simulink model "Autopilot_q_full_5may_new"  (R2020a)
settings: Solver=ode4  StartTime=0.0  StopTime=300  FixedStep=0.01  RelTol=1e-3
undefined symbols (not defined in the file or in its folder): Aero_cofficients, Atmosphere_pert, Atmospheric_model, Counter_sensor_model, Earth, error_global, flags_global, Guidance_Flags_global, INT_global, param_guidance, Payload_data, Plane_state_mode_finish_catcher_ftr_mode, Plane_state_mode_finish_catcher_fw_mode, Plane_state_mode_finish_catcher_q_mode, Plane_state_mode_finish_catcher_rtr_mode, Plane_state_store, propulsion_model, propulsion_model_int, Structural_data, Thrust_data_store, time_global, WGS84, Wind_data, Wind_model_int, Wind_pert_factor
libraries: simulink x33, aerolibactuator x15, cstblocks x3, aerolibatmos2 x2, aerolibfltsims x1, aerolibtransform2 x1, shared6dof x1
(part 7 of 10)

== matlab function Autopilot_q_full_5may_new/GUIDANCE/    MODE SWITCHER   &   PATH PLANNER   ==
  data: Time_global input; flags_global input; u_dot_d output; v_dot_d output; t input; Plane_state input; w_dot_d output; flags_global output; param_guidance output; param_guidance input; guidance_global input; INT_global input; error_global input; guidance_global output; INT_global output; error_global output; Wind_ned input; propulsion_data input; atmos_data input; wind_pert_factor input; propulsion_pert_factor input; structure_pert_factor input; atmos_pert_factor input; aero_coff_pert_factor input; data7 input; data8 input; data9 input; data10 input; data11 input; data12 input
function [u_dot_d,v_dot_d,w_dot_d,flags_global, param_guidance,guidance_global,INT_global,error_global] = fcn(Time_global, flags_global, t, Plane_state,param_guidance,guidance_global,INT_global,error_global, Wind_ned, propulsion_data, atmos_data, wind_pert_factor, propulsion_pert_factor, structure_pert_factor, atmos_pert_factor, aero_coff_pert_factor, data7, data8, data9, data10, data11, data12)

u_dot_d=0.0;
v_dot_d=0.0;
w_dot_d=0.0;

X_i_takeoff=guidance_global(1);  Y_i_takeoff=guidance_global(2);  Z_i_takeoff=guidance_global(3); X_f_takeoff=guidance_global(4); Y_f_takeoff=guidance_global(5); Z_f_takeoff=guidance_global(6);

X_i_hover=guidance_global(7); Y_i_hover=guidance_global(8); Z_i_hover=guidance_global(9); X_f_hover=guidance_global(10); Y_f_hover=guidance_global(11); Z_f_hover=guidance_global(12);

X_i_cruise=guidance_global(13); Y_i_cruise=guidance_global(14); Z_i_cruise=guidance_global(15); X_f_cruise=guidance_global(16); Y_f_cruise=guidance_global(17); Z_f_cruise=guidance_global(18);

X_i_circle=guidance_global(19); Y_i_circle=guidance_global(20); Z_i_circle=guidance_global(21); X_f_circle=guidance_global(22); Y_f_circle=guidance_global(23); Z_f_circle=guidance_global(24);

X_i_landing=guidance_global(25); Y_i_landing=guidance_global(26); Z_i_landing=guidance_global(27); X_f_landing=guidance_global(28); Y_f_landing=guidance_global(29); Z_f_landing=guidance_global(30);

X_f_forward_transition=guidance_global(31); Y_f_forward_transition=guidance_global(32); Z_f_forward_transition=guidance_global(33);

X_i_forward_transition=guidance_global(37); Y_i_forward_transition=guidance_global(38); Z_i_forward_transition=guidance_global(39);

X_f_reverse_transition=guidance_global(43); Y_f_reverse_transition=guidance_global(44); Z_f_reverse_transition=guidance_global(45);

X_i_reverse_transition=guidance_global(49); Y_i_reverse_transition=guidance_global(50); Z_i_reverse_transition=guidance_global(51);

INT_X=INT_global(1); INT_Y=INT_global(2); INT_Z=INT_global(3);

INT_vx=INT_global(4); INT_vy=INT_global(5); INT_vz=INT_global(6);

INT_phi=INT_global(7); INT_theta=INT_global(8); INT_psi=INT_global(9);

INT_p=INT_global(10); INT_q=INT_global(11); INT_r=INT_global(12);

INT_alpha=INT_global(13); INT_beta=INT_global(14);

R_circ=param_guidance(1);
cruise_speed=param_guidance(2);

lmt_pos=param_guidance(3); lmt_vel=param_guidance(4);


error_X_old=error_global(1); error_Y_old=error_global(2); error_Z_old=error_global(3);

error_vx_old=error_global(4); error_vy_old=error_global(5); error_vz_old=error_global(6);





limit_position_X=0.001;
limit_position_Y=0.001;
limit_position_Z=0.001;
limit_velocity_vx=0.001;
limit_velocity_vy=0.001;
limit_velocity_vz=0.001;

tf0=Time_global(1);
%% Initial lift off hover
tf1=Time_global(2);
%% Vertical Takeoff
tf2=Time_global(3);
%% Hover
tf3=Time_global(4);
%% Transition Forward
tf4=Time_global(5);
%% Cruise/circle or Fixed wing mode
tf5=Time_global(6);
%% Reverse Transition
tf6=Time_global(7);
%% Hover
tf7=Time_global(8);
%% Vertical Land
tf8 = Time_global(9);
%%

all_initial_check_ok=flags_global(1);
default_mode=flags_global(2);
quad_mode=flags_global(3);
Transition_mode=flags_global(4);
Fixed_wing_mode=flags_global(5);
fail_safe_mode=flags_global(6);
fail_safe_mode_hover=flags_global(7);
fail_safe_mode_land=flags_global(8);
fail_safe_mode_2=flags_global(9);
flag_initial_lift_off_hover = flags_global(10);
flag_vertical_takeoff = flags_global(11);
flag_hover_mode = flags_global(12);
flag_circle_mode =  flags_global(13);
flag_cruise_mode = flags_global(14);
flag_vertical_landing = flags_global(15);

one_time_initial_lift_off_hover = flags_global(16);
one_time_initial_vertical_takeoff = flags_global(17);
one_time_initial_hover_mode = flags_global(18);
one_time_initial_cruise_mode = flags_global(19);
one_time_initial_circle_mode = flags_global(20);
one_time_initial_vertical_landing = flags_global(21);

flag_brake_mode=flags_global(22);

flag_forward_transition=flags_global(23);
flag_reverse_transition=flags_global(24);

one_time_initial_flag_forward_transition = flags_global(25);
one_time_initial_flag_reverse_transition = flags_global(26);


if ((t>=tf0)&&(t<tf1))
    quad_mode=1;
    Transition_mode=0;
    Fixed_wing_mode=0;
    flag_initial_lift_off_hover=1;
    flag_vertical_takeoff=0;
    flag_hover_mode=0;
    flag_cruise_mode=0;
    flag_circle_mode=0;
    flag_vertical_landing=0;
    flag_forward_transition=0;
    flag_reverse_transition=0;
    flag_brake_mode=0;
   % one_time_initial_lift_off_hover = 1;
    one_time_initial_vertical_takeoff =1;
    one_time_initial_hover_mode = 1;
    one_time_initial_cruise_mode = 1;
    one_time_initial_circle_mode = 1;
    one_time_initial_vertical_landing =1;
    one_time_initial_flag_forward_transition = 1;
    one_time_initial_flag_reverse_transition =1 ;

    
end

if ((t>=tf1)&&(t<tf2))
    quad_mode=1;
    Transition_mode=0;
    Fixed_wing_mode=0;
    flag_initial_lift_off_hover=0;
    flag_vertical_takeoff=1;
    flag_hover_mode=0;
    flag_cruise_mode=0;
    flag_circle_mode=0;
    flag_vertical_landing=0;
    flag_forward_transition=0;
    flag_reverse_transition=0;
    flag_brake_mode=0;
    one_time_initial_lift_off_hover = 1;
    %one_time_initial_vertical_takeoff =1;
    one_time_initial_hover_mode = 1;
    one_time_initial_cruise_mode = 1;
    one_time_initial_circle_mode = 1;
    one_time_initial_vertical_landing =1;
    one_time_initial_flag_forward_transition = 1;
    one_time_initial_flag_reverse_transition =1 ;
end

if ((t>=tf2)&&(t<tf3))
    quad_mode=1;
    Transition_mode=0;
    Fixed_wing_mode=0;
    flag_initial_lift_off_hover=0;
    flag_vertical_takeoff=0;
    flag_hover_mode=1;
    flag_cruise_mode=0;
    flag_circle_mode=0;
    flag_vertical_landing=0;
    flag_forward_transition=0;
    flag_reverse_transition=0;
    flag_brake_mode=0;
    one_time_initial_lift_off_hover = 1;
    one_time_initial_vertical_takeoff =1;
    %one_time_initial_hover_mode = 1;
    one_time_initial_cruise_mode = 1;
    one_time_initial_circle_mode = 1;
    one_time_initial_vertical_landing =1;
    one_time_initial_flag_forward_transition = 1;
    one_time_initial_flag_reverse_transition =1 ;
end

if ((t>=tf3)&&(t<tf4))
    quad_mode=0;
    Transition_mode=1;
    Fixed_wing_mode=0;
    flag_forward_transition=1;
    flag_reverse_transition=0;
    flag_initial_lift_off_hover=0;
    flag_vertical_takeoff=0;
    flag_hover_mode=0;
    flag_cruise_mode=0;
    flag_circle_mode=0;
    flag_vertical_landing=0;
    flag_brake_mode=0;
    one_time_initial_lift_off_hover = 1;
    one_time_initial_vertical_takeoff =1;
    one_time_initial_hover_mode = 1;
    one_time_initial_cruise_mode = 1;
    one_time_initial_circle_mode = 1;
    one_time_initial_vertical_landing =1;
    %one_time_initial_flag_forward_transition = 1;
    one_time_initial_flag_reverse_transition =1 ;
end

if ((t>=tf4)&&(t<tf5))
    quad_mode=0;
    Transition_mode=0;
    Fixed_wing_mode=1;
    flag_cruise_mode=1;
    flag_circle_mode=0;
    flag_initial_lift_off_hover=0;
    flag_vertical_takeoff=0;
    flag_hover_mode=0;
    flag_vertical_landing=0;
    flag_forward_transition=0;
    flag_reverse_transition=0;
    flag_brake_mode=0;
    one_time_initial_lift_off_hover = 1;
    one_time_initial_vertical_takeoff =1;
    one_time_initial_hover_mode = 1;
    %one_time_initial_cruise_mode = 1;
    one_time_initial_circle_mode = 1;
    one_time_initial_vertical_landing =1;
    one_time_initial_flag_forward_transition = 1;
    one_time_initial_flag_reverse_transition =1 ;
end

if ((t>=tf5)&&(t<tf6))
    quad_mode=0;
    Transition_mode=1;
    Fixed_wing_mode=0;
    flag_forward_transition=0;
    flag_reverse_transition=1;
    flag_initial_lift_off_hover=0;
    flag_vertical_takeoff=0;
    flag_hover_mode=0;
    flag_cruise_mode=0;
    flag_circle_mode=0;
    flag_vertical_landing=0;
    flag_brake_mode=0;
    one_time_initial_lift_off_hover = 1;
    one_time_initial_vertical_takeoff =1;
    one_time_initial_hover_mode = 1;
    one_time_initial_cruise_mode = 1;
    one_time_initial_circle_mode = 1;
    one_time_initial_vertical_landing =1;
    one_time_initial_flag_forward_transition = 1;
   % one_time_initial_flag_reverse_transition =1 ;

end

if ((t>=tf6)&&(t<tf7))
    quad_mode=1;
    Transition_mode=0;
    Fixed_wing_mode=0;
    flag_initial_lift_off_hover=0;
    flag_vertical_takeoff=0;
    flag_hover_mode=1;
    flag_cruise_mode=0;
    flag_circle_mode=0;
    flag_vertical_landing=0;
    flag_forward_transition=0;
    flag_reverse_transition=0;
    flag_brake_mode=0;
    %one_time_initial_lift_off_hover = 1;
    one_time_initial_vertical_takeoff =1;
    one_time_initial_hover_mode = 1;
    one_time_initial_cruise_mode = 1;
    one_time_initial_circle_mode = 1;
    one_time_initial_vertical_landing =1;
    one_time_initial_flag_forward_transition = 1;
    one_time_initial_flag_reverse_transition =1 ;
end

if ((t>=tf7)&&(t<tf8))
    quad_mode=1;
    Transition_mode=0;
    Fixed_wing_mode=0;
    flag_initial_lift_off_hover=0;
    flag_vertical_takeoff=0;
    flag_hover_mode=0;
    flag_cruise_mode=0;
    flag_circle_mode=0;
    flag_vertical_landing=1;
    flag_forward_transition=0;
    flag_reverse_transition=0;
    flag_brake_mode=0;
    one_time_initial_lift_off_hover = 1;
    one_time_initial_vertical_takeoff =1;
    one_time_initial_hover_mode = 1;
    one_time_initial_cruise_mode = 1;
    one_time_initial_circle_mode = 1;
    %one_time_initial_vertical_landing =1;
    one_time_initial_flag_forward_transition = 1;
    one_time_initial_flag_reverse_transition =1 ;
end

u=Plane_state(1);
v=Plane_state(2);
w=Plane_state(3);
p=Plane_state(4);
q=Plane_state(5);
r=Plane_state(6);
phi=Plane_state(7);
theta=Plane_state(8);
psi=Plane_state(9);
X=Plane_state(10);
Y=Plane_state(11);
Z=Plane_state(12);

R_v_v1=[cos(psi) sin(psi) 0; -sin(psi) cos(psi) 0; 0 0 1];
R_v1_v2=[cos(theta) 0 -sin(theta) ;0 1 0; sin(theta) 0 cos(theta)];
R_v2_b=[1 0 0;0 cos(phi) sin(phi) ;0 -sin(phi) cos(phi)];
R_v_b=R_v2_b*R_v1_v2*R_v_v1;



V_wind_bd=R_v_b*[Wind_ned(1);Wind_ned(2);Wind_ned(3)];

ppp = [u-V_wind_bd(1); v; w];
u_r=ppp(1);
v_r=ppp(2);
w_r=ppp(3);

V=sqrt(u_r^2+v_r^2+w_r^2);


%%
%%%%%%%%%%%%%%%%%%%%%%%%%%%%%%%%%%%%%%%%%%%%%%%%%%%%%%%%%%%%%%%%%%%%%%%%%%%%%%%%%%%%%%%%%%%%%%%%%%%%%%%%%%%%%%%%%%%%%%%%%%%%
%%%%%%%%%%%%%%%%%%%%%%%%%%%%%%%%%%%%%%%%%%%%%%%%%%%%%%%%%%%%%%%%%%%%%%%%%%%%%%%%%%%%%%%%%%%%%%%%%%%%%%%%%%%%%%%%%%%%%%%%%%%%
%%%%%%%%%%%%%%%%%%%%%%%%%%%%%%%%%%%%%%%%%%%%%%%%%%%%%%%%%%%%%%%%%%%%%%%%%%%%%%%%%%%%%%%%%%%%%%%%%%%%%%%%%%%%%%%%%%%%%%%%%%%%
if (default_mode==1)
    X_d=X;
    Y_d=Y;
    Z_d=Z;
    u_d=0.0;
    v_d=0.0;
    w_d=0.0;
    
    
    Kp_vx= 0.1*4.0*3.0;  
    Kp_vy= 0.1*4.0*3.0;    
    Kp_vz= 6.0;            
    
    error_vx = (u_d-u);
    error_vy = (v_d-v);
    error_vz = (w_d-w);
    
    u_dot_d = Kp_vx*(error_vx) ;  
    v_dot_d = Kp_vy*(error_vy) ;
    w_dot_d = Kp_vz*(error_vz) ;
end
%%
if (fail_safe_mode==0)
    
if (flag_initial_lift_off_hover==1)
    if (one_time_initial_hover_mode==1)
        X_i_hover=X;
        Y_i_hover=Y;
        Z_i_hover=Z;
        
        X_f_hover=X_i_hover;
        Y_f_hover=Y_i_hover;
        Z_f_hover=Z_i_hover;
        
        INT_X=0;INT_Y=0;INT_Z=0;
        INT_vx=0;INT_vy=0;INT_vz=0;
        INT_alpha=0;INT_beta=0;
        
        INT_phi=0;INT_theta=0;INT_psi=0;
        INT_p=0;INT_q=0;INT_r=0;
        
        one_time_initial_hover_mode=0;
    end
    
    X_d=X_f_hover;
    Y_d=Y_f_hover;
    Z_d=Z_f_hover;
    
    Kp_X=0.1*2.0;           Ki_X= 0.0;                Kd_X=0.0;
    Kp_Y=0.1*2.0;           Ki_Y= 0.0;                Kd_Y=0.0;
    Kp_Z=0.1;               Ki_Z=Kp_Z/10.0;           Kd_Z=0.0;
    
    Kp_vx= 0.1*2.0*3.0;     Ki_vx=0.0;                Kd_vx=0.0;
    Kp_vy= 0.1*2.0*3.0;     Ki_vy=0.0;                Kd_vy=0.0;
    Kp_vz= 0.3;             Ki_vz=0.01;               Kd_vz=0.0;
    
    
    error_X = (X_d-X);
    error_Y = (Y_d-Y);
    error_Z = (Z_d-Z);
    
    if(lmt_pos==1)
        
        if(abs(error_X)<limit_position_X)
            
            error_X=0.0;
        end
        if(abs(error_Y)<limit_position_Y)
            
            error_Y=0.0;
        end
        if(abs(error_Z)<limit_position_Z)
            
            error_Z=0.0;
        end
    end
    
    INT_X = INT_X + 0.01*(error_X);
    INT_Y = INT_Y + 0.01*(error_Y);
    INT_Z = INT_Z + 0.01*(error_Z);
    
    U_d = Kp_X*(error_X) +  Ki_X*(INT_X) + Kd_X*(error_X-error_X_old);
    V_d = Kp_Y*(error_Y) +  Ki_Y*(INT_Y) + Kd_Y*(error_Y-error_Y_old);
    W_d = Kp_Z*(error_Z) +  Ki_Z*(INT_Z) + Kd_Z*(error_Z-error_Z_old);
    
    temp_3X1=R_v_b*[U_d;V_d;W_d];
    
    u_d=temp_3X1(1);
    v_d=temp_3X1(2);
    w_d=temp_3X1(3);
    
    error_X_old=error_X;
    error_Y_old=error_Y;
    error_Z_old=error_Z;
    
    error_vx = (u_d-u);
    error_vy = (v_d-v);
    error_vz = (w_d-w);
    
    if(lmt_vel==1)
        if(abs(error_vx)<limit_velocity_vx)
            error_vx=0.0;
        end
        if(abs(error_vy)<limit_velocity_vy)
            error_vy=0.0;
        end
        if(abs(error_vz)<limit_velocity_vz)
            error_vz=0.0;
        end
    end
    
    INT_vx= INT_vx + 0.01*(error_vx);
    INT_vy= INT_vy + 0.01*(error_vy);
    INT_vz= INT_vz + 0.01*(error_vz);
    
    u_dot_d = Kp_vx*(error_vx)   +    Ki_vx*(INT_vx)  +   Kd_vx*(error_vx-error_vx_old);
    v_dot_d = Kp_vy*(error_vy)   +    Ki_vy*(INT_vy)  +   Kd_vy*(error_vy-error_vy_old);
    w_dot_d = Kp_vz*(error_vz)   +    Ki_vz*(INT_vz)  +   Kd_vz*(error_vz-error_vz_old);
    
    error_vx_old=error_vx;
    error_vy_old=error_vy;
    error_vz_old=error_vz;
    
end

if (flag_vertical_takeoff==1)
    if (one_time_initial_vertical_takeoff==1)
        
        X_i_takeoff = X;
        Y_i_takeoff = Y;
        Z_i_takeoff = Z;
        
        X_f_takeoff = X_i_takeoff;
        Y_f_takeoff = Y_i_takeoff;
        Z_f_takeoff = Z_i_takeoff-50.0;
        
        INT_X=0;INT_Y=0;INT_Z=0;
        INT_vx=0;INT_vy=0;INT_vz=0;
        
        INT_alpha=0;INT_beta=0;
        
        INT_phi=0;INT_theta=0;INT_psi=0;
        INT_p=0;INT_q=0;INT_r=0;
        
        one_time_initial_vertical_takeoff=0;
        one_time_initial_hover_mode=1;
    end
    
    X_d=X_f_takeoff;
    Y_d=Y_f_takeoff;
    Z_d=Z_i_takeoff + 2*(Z_f_takeoff-Z_i_takeoff)*(t-tf1)/(tf2-tf1) +(Z_i_takeoff-Z_f_takeoff)*((t-tf1)^2)/((tf2-tf1)^2) ;
   if t>tf2
       Z_d = Z_f_takeoff;
    end
    Kp_X=0.1*4.0;           Ki_X= 0.0;                Kd_X=0.0;
    Kp_Y=0.1*4.0;           Ki_Y= 0.0;                Kd_Y=0.0;
    Kp_Z=2.0;              Ki_Z=0.1;           Kd_Z=0.0;
    
    Kp_vx= 0.1*4.0*3.0;     Ki_vx=0.0;                Kd_vx=0.0;
    Kp_vy= 0.1*4.0*3.0;     Ki_vy=0.0;                Kd_vy=0.0;
    Kp_vz= 6.0;             Ki_vz=0.0*0.001;               Kd_vz=0.0;
    
    
    error_X = (X_d-X);
    error_Y = (Y_d-Y);
    error_Z = (Z_d-Z);
    
    if(lmt_pos==1)
        
        if(abs(error_X)<limit_position_X)
            
            error_X=0.0;
        end
        if(abs(error_Y)<limit_position_Y)
            
            error_Y=0.0;
        end
        if(abs(error_Z)<limit_position_Z)
            
            error_Z=0.0;
        end
    end
    
    INT_X = INT_X + 0.01*(error_X);
    INT_Y = INT_Y + 0.01*(error_Y);
    INT_Z = INT_Z + 0.01*(error_Z);
    
    U_d = Kp_X*(error_X) +  Ki_X*(INT_X) + Kd_X*(error_X-error_X_old);
    V_d = Kp_Y*(error_Y) +  Ki_Y*(INT_Y) + Kd_Y*(error_Y-error_Y_old);
    W_d = Kp_Z*(error_Z) +  Ki_Z*(INT_Z) + Kd_Z*(error_Z-error_Z_old);
    
    temp_3X1=R_v_b*[U_d;V_d;W_d];
    
    u_d=temp_3X1(1);
    v_d=temp_3X1(2);
    w_d=temp_3X1(3);
    error_X_old=error_X;
    error_Y_old=error_Y;
    error_Z_old=error_Z;
    
    error_vx = (u_d-u);
    error_vy = (v_d-v);
    error_vz = (w_d-w);
    
    if(lmt_vel==1)
        if(abs(error_vx)<limit_velocity_vx)
            error_vx=0.0;
        end
        if(abs(error_vy)<limit_velocity_vy)
            error_vy=0.0;
        end
        if(abs(error_vz)<limit_velocity_vz)
            error_vz=0.0;
        end
    end
    
    INT_vx= INT_vx + 0.01*(error_vx);
    INT_vy= INT_vy + 0.01*(error_vy);
    INT_vz= INT_vz + 0.01*(error_vz);
    
    u_dot_d = Kp_vx*(error_vx)   +    Ki_vx*(INT_vx)  +   Kd_vx*(error_vx-error_vx_old);
    v_dot_d = Kp_vy*(error_vy)   +    Ki_vy*(INT_vy)  +   Kd_vy*(error_vy-error_vy_old);
    w_dot_d = Kp_vz*(error_vz)   +    Ki_vz*(INT_vz)  +   Kd_vz*(error_vz-error_vz_old);
    
    error_vx_old=error_vx;
    error_vy_old=error_vy;
    error_vz_old=error_vz;

end

if (flag_hover_mode==1)
    if (one_time_initial_hover_mode==1)
        X_i_hover=X;
        Y_i_hover=Y;
        Z_i_hover=Z;
        
        X_f_hover = X_i_hover;
        Y_f_hover = Y_i_hover;
        Z_f_hover = Z_i_hover;
        
        INT_X=0;INT_Y=0;INT_Z=0;
        INT_vx=0;INT_vy=0;INT_vz=0;
        INT_alpha=0;INT_beta=0;
        
        INT_phi=0;INT_theta=0;INT_psi=0;
        INT_p=0;INT_q=0;INT_r=0;
        
        one_time_initial_hover_mode=0;
    end
    
    X_d=X_i_hover;
    Y_d=Y_i_hover;
    Z_d=Z_i_hover;
    
    Kp_X=0.1*4.0;           Ki_X= 0.0;                Kd_X=0.0;
    Kp_Y=0.1*4.0;           Ki_Y= 0.0;                Kd_Y=0.0;
    Kp_Z=2.0;               Ki_Z=0.01;                Kd_Z=0.0;
    
    Kp_vx= 0.1*4.0*3.0;     Ki_vx=0.0;                Kd_vx=0.0;
    Kp_vy= 0.1*4.0*3.0;     Ki_vy=0.0;                Kd_vy=0.0;
    Kp_vz= 6.0;             Ki_vz=0.01*0;             Kd_vz=0.0;
    
    
    error_X = (X_d-X);
    error_Y = (Y_d-Y);
    error_Z = (Z_d-Z);
    
    if(lmt_pos==1)
        
        if(abs(error_X)<limit_position_X)
            
            error_X=0.0;
        end
        if(abs(error_Y)<limit_position_Y)
            
            error_Y=0.0;
        end
        if(abs(error_Z)<limit_position_Z)
            
            error_Z=0.0;
        end
    end
    
    INT_X = INT_X + 0.01*(error_X);
    INT_Y = INT_Y + 0.01*(error_Y);
    INT_Z = INT_Z + 0.01*(error_Z);
    
    U_d = Kp_X*(error_X) +  Ki_X*(INT_X) + Kd_X*(error_X-error_X_old);
    V_d = Kp_Y*(error_Y) +  Ki_Y*(INT_Y) + Kd_Y*(error_Y-error_Y_old);
    W_d = Kp_Z*(error_Z) +  Ki_Z*(INT_Z) + Kd_Z*(error_Z-error_Z_old);
    
    temp_3X1=R_v_b*[U_d;V_d;W_d];
    
    u_d=temp_3X1(1);
    v_d=temp_3X1(2);
    w_d=temp_3X1(3);
    error_X_old=error_X;
    error_Y_old=error_Y;
    error_Z_old=error_Z;
    
    error_vx = (u_d-u);
    error_vy = (v_d-v);
    error_vz = (w_d-w);
    
    if(lmt_vel==1)
        if(abs(error_vx)<limit_velocity_vx)
            error_vx=0.0;
        end
        if(abs(error_vy)<limit_velocity_vy)
            error_vy=0.0;
        end
        if(abs(error_vz)<limit_velocity_vz)
            error_vz=0.0;
        end
    end
    
    INT_vx= INT_vx + 0.01*(error_vx);
    INT_vy= INT_vy + 0.01*(error_vy);
    INT_vz= INT_vz + 0.01*(error_vz);
    
    u_dot_d = Kp_vx*(error_vx)   +    Ki_vx*(INT_vx)  +   Kd_vx*(error_vx-error_vx_old);
    v_dot_d = Kp_vy*(error_vy)   +    Ki_vy*(INT_vy)  +   Kd_vy*(error_vy-error_vy_old);
    w_dot_d = Kp_vz*(error_vz)   +    Ki_vz*(INT_vz)  +   Kd_vz*(error_vz-error_vz_old);
    
    error_vx_old=error_vx;
    error_vy_old=error_vy;
    error_vz_old=error_vz;
    
end

if (flag_forward_transition==1)
    if (one_time_initial_flag_forward_transition==1)
        X_i_forward_transition=X;
        Y_i_forward_transition=Y;
        Z_i_forward_transition=Z;
        
        X_f_forward_transition=X_i_forward_transition;
        Y_f_forward_transition=Y_i_forward_transition;
        Z_f_forward_transition=Z_i_forward_transition;
        
        INT_X=0;INT_Y=0;INT_Z=0;
        INT_vx=0;INT_vy=0;INT_vz=0;
        INT_alpha=0;INT_beta=0;
        
        INT_phi=0;INT_theta=0;INT_psi=0;
        INT_p=0;INT_q=0;INT_r=0;
        
        one_time_initial_flag_forward_transition=0;
    end
    

    Kp_Z=2.0;               Ki_Z=0.01;                Kd_Z=0.0;
    
    Kp_vx= 0.1*4.0*3.0;     Ki_vx=0.0;                Kd_vx=0.0;
    Kp_vy= 0.1*4.0*3.0;     Ki_vy=0.0;                Kd_vy=0.0;
    Kp_vz= 6.0;             Ki_vz=0.0;                Kd_vz=0.0;
    
    X_d=X;
    Y_d=Y;
    Z_d= Z_f_forward_transition;
    
    error_X = (X_d-X);
    error_Y = (Y_d-Y);
    error_Z = (Z_d-Z);
    
    if(lmt_pos==1)
        
        if(abs(error_X)<limit_position_X)
            
            error_X=0.0;
        end
        if(abs(error_Y)<limit_position_Y)
            
            error_Y=0.0;
        end
        if(abs(error_Z)<limit_position_Z)
            
            error_Z=0.0;
        end
    end
    
    INT_X = INT_X + 0.01*(error_X);
    INT_Y = INT_Y + 0.01*(error_Y);
    INT_Z = INT_Z + 0.01*(error_Z);
    
    % U_d = Kp_X*(error_X) +  Ki_X*(INT_X) + Kd_X*(error_X-error_X_old);
    V_X_i_cruise=0.0;
    V_X_f_cruise=cruise_speed;
    
    U_d_1= (V_X_i_cruise + 2*(V_X_f_cruise-V_X_i_cruise)*(t-tf3)/(tf4-tf3) -(V_X_f_cruise-V_X_i_cruise)*((t-tf3)^2)/((tf4-tf3)^2)) ;
    
    if t>tf4
        U_d_1 = cruise_speed;
    end
    % V_d = Kp_Y*(error_Y) +  Ki_Y*(INT_Y) + Kd_Y*(error_Y-error_Y_old);
    V_d_1=0.0;
    
    W_d_1 = Kp_Z*(error_Z) +  Ki_Z*(INT_Z) + Kd_Z*(error_Z-error_Z_old);

    temp_3X1=R_v2_b*R_v1_v2*[U_d_1;V_d_1;W_d_1];
    
    u_d = temp_3X1(1) ;
    v_d = temp_3X1(2) ;
    w_d = temp_3X1(3) ;
	
    
    error_X_old=error_X;
    error_Y_old=error_Y;
    error_Z_old=error_Z;
    
    error_vx = (u_d-u_r);
    error_vy = (v_d-v_r);
    error_vz = (w_d-w_r);
    
    if(lmt_vel==1)
        if(abs(error_vx)<limit_velocity_vx)
            error_vx=0.0;
        end
        if(abs(error_vy)<limit_velocity_vy)
            error_vy=0.0;
        end
        if(abs(error_vz)<limit_velocity_vz)
            error_vz=0.0;
        end
    end
    
    INT_vx= INT_vx + 0.01*(error_vx);
    INT_vy= INT_vy + 0.01*(error_vy);
    INT_vz= INT_vz + 0.01*(error_vz);
    
    u_dot_d = Kp_vx*(error_vx)   +    Ki_vx*(INT_vx)  +   Kd_vx*(error_vx-error_vx_old);
    v_dot_d = Kp_vy*(error_vy)   +    Ki_vy*(INT_vy)  +   Kd_vy*(error_vy-error_vy_old);
    w_dot_d = Kp_vz*(error_vz)   +    Ki_vz*(INT_vz)  +   Kd_vz*(error_vz-error_vz_old);
    
    error_vx_old=error_vx;
    error_vy_old=error_vy;
    error_vz_old=error_vz;
    
end


if (flag_circle_mode==1)
    if (one_time_initial_circle_mode==1)
        X_i_circle=X;
        Y_i_circle=Y;
        Z_i_circle=Z;
        
        X_f_circle=X_i_circle;
        Y_f_circle=Y_i_circle;
        Z_f_circle=Z_i_circle;
        one_time_initial_circle_mode=0;
        
        INT_X=0;INT_Y=0;INT_Z=0;
        INT_vx=0;INT_vy=0;INT_vz=0;
        INT_alpha=0;INT_beta=0;
        
        INT_phi=0;INT_theta=0;INT_psi=0;
        INT_p=0;INT_q=0;INT_r=0;
    end
    X_d = R_circ*sin((t-tf4)*((2*3.1415)/(tf5-tf4))) + X_i_circle;
    Y_d = R_circ*cos((t-tf4)*((2*3.1415)/(tf5-tf4))) + Y_i_circle - R_circ;
    Z_d = Z_f_circle;
    
    Kp_X=0.1*4.0;           Ki_X=0.00;                 Kd_X=0.0;
    Kp_Y=0.1*4.0;           Ki_Y=0.00;                 Kd_Y=0.0;
    Kp_Z=2.0;               Ki_Z=0.01;                 Kd_Z=0.0;
    
    Kp_vx= 0.1*4.0*3.0;     Ki_vx=0.00;                Kd_vx=0.0;
    Kp_vy= 0.1*4.0*3.0;     Ki_vy=0.00;                Kd_vy=0.0;
    Kp_vz= 6.0;             Ki_vz=0.00;                Kd_vz=0.0;
    
    
    error_X = (X_d-X);
    error_Y = (Y_d-Y);
    error_Z = (Z_d-Z);
    
    if(lmt_pos==1)
        
        if(abs(error_X)<limit_position_X)
            
            error_X=0.0;
        end
        if(abs(error_Y)<limit_position_Y)
            
            error_Y=0.0;
        end
        if(abs(error_Z)<limit_position_Z)
            
            error_Z=0.0;
        end
    end
    
    INT_X = INT_X + 0.01*(error_X);
    INT_Y = INT_Y + 0.01*(error_Y);
    INT_Z = INT_Z + 0.01*(error_Z);
    
    U_d = Kp_X*(error_X) +  Ki_X*(INT_X) + Kd_X*(error_X-error_X_old);
    V_d = Kp_Y*(error_Y) +  Ki_Y*(INT_Y) + Kd_Y*(error_Y-error_Y_old);
    W_d = Kp_Z*(error_Z) +  Ki_Z*(INT_Z) + Kd_Z*(error_Z-error_Z_old);
    
    temp_3X1=R_v_b*[U_d;V_d;W_d];
    
    u_d=temp_3X1(1);
    v_d=temp_3X1(2);
    w_d=temp_3X1(3);
    error_X_old=error_X;
    error_Y_old=error_Y;
    error_Z_old=error_Z;
    
    error_vx = (u_d-u_r);% wind longitudinal component considered
    error_vy = (v_d-v_r);
    error_vz = (w_d-w_r);
    
    if(lmt_vel==1)
        if(abs(error_vx)<limit_velocity_vx)
            error_vx=0.0;
        end
        if(abs(error_vy)<limit_velocity_vy)
            error_vy=0.0;
        end
        if(abs(error_vz)<limit_velocity_vz)
            error_vz=0.0;
        end
    end
    
    INT_vx= INT_vx + 0.01*(error_vx);
    INT_vy= INT_vy + 0.01*(error_vy);
    INT_vz= INT_vz + 0.01*(error_vz);
    
    u_dot_d = Kp_vx*(error_vx)   +    Ki_vx*(INT_vx)  +   Kd_vx*(error_vx-error_vx_old);
    v_dot_d = Kp_vy*(error_vy)   +    Ki_vy*(INT_vy)  +   Kd_vy*(error_vy-error_vy_old);
    w_dot_d = Kp_vz*(error_vz)   +    Ki_vz*(INT_vz)  +   Kd_vz*(error_vz-error_vz_old);
    
    error_vx_old=error_vx;
    error_vy_old=error_vy;
    error_vz_old=error_vz;
    
end

if (flag_cruise_mode==1)
    if (one_time_initial_cruise_mode==1)
        X_i_cruise=X;
        Y_i_cruise=Y;
        Z_i_cruise=Z;
        
        X_f_cruise=X_i_cruise;
        Y_f_cruise=Y_i_cruise;
        Z_f_cruise=Z_i_cruise;
        
        INT_X=0;INT_Y=0;INT_Z=0;
        INT_vx=0;INT_vy=0;INT_vz=0;
        
        INT_alpha=0;INT_beta=0;
        
        INT_phi=0;INT_theta=0;INT_psi=0;
        INT_p=0;INT_q=0;INT_r=0;
        
        one_time_initial_cruise_mode=0;
        
    end
    
    X_d=X;
    Y_d=Y;
    Z_d= Z_f_cruise;
    
    
 
    Kp_Z=2.0;               Ki_Z=0.01;           Kd_Z=0.0;
    
    Kp_vx= 0.1*4.0*3.0;     Ki_vx=0.0;                Kd_vx=0.0;
    Kp_vy= 0.1*4.0*3.0;     Ki_vy=0.0;                Kd_vy=0.0;
    Kp_vz= 6.0;             Ki_vz=0.0;               Kd_vz=0.0;
    
    
    error_X = (X_d-X);
    error_Y = (Y_d-Y);
    error_Z = (Z_d-Z);
    
    if(lmt_pos==1)
        
        if(abs(error_X)<limit_position_X)
            
            error_X=0.0;
        end
        if(abs(error_Y)<limit_position_Y)
            
            error_Y=0.0;
        end
        if(abs(error_Z)<limit_position_Z)
            
            error_Z=0.0;
        end
    end
    
    INT_X = INT_X + 0.01*(error_X);
    INT_Y = INT_Y + 0.01*(error_Y);
    INT_Z = INT_Z + 0.01*(error_Z);
    
    
    U_d_1= cruise_speed;
    
    % V_d = Kp_Y*(error_Y) +  Ki_Y*(INT_Y) + Kd_Y*(error_Y-error_Y_old);
    V_d_1=0.0;
    
    W_d_1 = Kp_Z*(error_Z) +  Ki_Z*(INT_Z) + Kd_Z*(error_Z-error_Z_old);

    temp_3X1=R_v2_b*R_v1_v2*[U_d_1;V_d_1;W_d_1];
    
    u_d = temp_3X1(1) ;
    v_d = temp_3X1(2) ;
    w_d = temp_3X1(3) ;
    
    error_X_old=error_X;
    error_Y_old=error_Y;
    error_Z_old=error_Z;
    
    error_vx = (u_d-u_r);% wind longitudinal component considered
    error_vy = (v_d-v_r);
    error_vz = (w_d-w_r);
    
    if(lmt_vel==1)
        if(abs(error_vx)<limit_velocity_vx)
            error_vx=0.0;
        end
        if(abs(error_vy)<limit_velocity_vy)
            error_vy=0.0;
        end
        if(abs(error_vz)<limit_velocity_vz)
            error_vz=0.0;
        end
    end
    
    INT_vx= INT_vx + 0.01*(error_vx);
    INT_vy= INT_vy + 0.01*(error_vy);
    INT_vz= INT_vz + 0.01*(error_vz);
    
    u_dot_d = Kp_vx*(error_vx)   +    Ki_vx*(INT_vx)  +   Kd_vx*(error_vx-error_vx_old);
    v_dot_d = Kp_vy*(error_vy)   +    Ki_vy*(INT_vy)  +   Kd_vy*(error_vy-error_vy_old);
    w_dot_d = Kp_vz*(error_vz)   +    Ki_vz*(INT_vz)  +   Kd_vz*(error_vz-error_vz_old);
    
    error_vx_old=error_vx;
    error_vy_old=error_vy;
    error_vz_old=error_vz;
    
end

if (flag_reverse_transition==1)
    if (one_time_initial_flag_reverse_transition==1)
        X_i_reverse_transition=X;
        Y_i_reverse_transition=Y;
        Z_i_reverse_transition=Z;
        
        X_f_reverse_transition=X_i_reverse_transition;
        Y_f_reverse_transition=Y_i_reverse_transition;
        Z_f_reverse_transition=Z_i_reverse_transition;
        
        INT_X=0;INT_Y=0;INT_Z=0;
        INT_vx=0;INT_vy=0;INT_vz=0;
        INT_alpha=0;INT_beta=0;
        
        INT_phi=0;INT_theta=0;INT_psi=0;
        INT_p=0;INT_q=0;INT_r=0;
        
        one_time_initial_flag_reverse_transition=0;
    end
    
    Kp_X=0.1*4.0;           Ki_X=0.00;                 Kd_X=0.0;
    Kp_Y=0.1*4.0;           Ki_Y=0.00;                 Kd_Y=0.0;
    Kp_Z=2.0;               Ki_Z=0.01;                 Kd_Z=0.0;
    
    Kp_vx= 0.1*4.0*3.0;     Ki_vx=0.00;                Kd_vx=0.0;
    Kp_vy= 0.1*4.0*3.0;     Ki_vy=0.00;                Kd_vy=0.0;
    Kp_vz= 6.0;             Ki_vz=0.00;                Kd_vz=0.0;
    
    X_d=X;
    Y_d=Y;
    Z_d= Z_f_cruise;
    
    error_X = (X_d-X);
    error_Y = (Y_d-Y);
    error_Z = (Z_d-Z);
    
    if(lmt_pos==1)
        
        if(abs(error_X)<limit_position_X)
            
            error_X=0.0;
        end
        if(abs(error_Y)<limit_position_Y)
            
            error_Y=0.0;
        end
        if(abs(error_Z)<limit_position_Z)
            
            error_Z=0.0;
        end
    end
    
    INT_X = INT_X + 0.01*(error_X);
    INT_Y = INT_Y + 0.01*(error_Y);
    INT_Z = INT_Z + 0.01*(error_Z);
    
    V_X_i_cruise=cruise_speed;
    V_X_f_cruise=0.0;
    % U_d = Kp_X*(error_X) +  Ki_X*(INT_X) + Kd_X*(error_X-error_X_old);
    U_d_1=V_X_i_cruise + 2*(V_X_f_cruise-V_X_i_cruise)*(t-tf5)/(tf6-tf5) -(V_X_f_cruise-V_X_i_cruise)*((t-tf5)^2)/((tf6-tf5)^2) ;
    if t>tf6
        U_d_1 = V_X_f_cruise;
    end
    % V_d = Kp_Y*(error_Y) +  Ki_Y*(INT_Y) + Kd_Y*(error_Y-error_Y_old);
    V_d_1=0.0;
    W_d_1 = Kp_Z*(error_Z) +  Ki_Z*(INT_Z) + Kd_Z*(error_Z-error_Z_old);

    
    temp_3X1=R_v2_b*R_v1_v2*[U_d_1;V_d_1;W_d_1];
    
    u_d = temp_3X1(1) ;
    v_d = temp_3X1(2) ;
    w_d = temp_3X1(3) ;
    %u_d=temp_3X1(1);

   % u_d = V_X_i_cruise + 2*(V_X_f_cruise-V_X_i_cruise)*(t-tf5)/(tf6-tf5) -(V_X_f_cruise-V_X_i_cruise)*((t-tf5)^2)/((tf6-tf5)^2) ;
	
   % v_d=temp_3X1(2);
%     v_d=0.0;
%     w_d=temp_3X1(3);
    
    error_X_old=error_X;
    error_Y_old=error_Y;
    error_Z_old=error_Z;
    
    error_vx = (u_d-u_r);% wind longitudinal component considered
    error_vy = (v_d-v_r);
    error_vz = (w_d-w_r);
    
    if(lmt_vel==1)
        if(abs(error_vx)<limit_velocity_vx)
            error_vx=0.0;
        end
        if(abs(error_vy)<limit_velocity_vy)
            error_vy=0.0;
        end
        if(abs(error_vz)<limit_velocity_vz)
            error_vz=0.0;
        end
    end
    
    INT_vx= INT_vx + 0.01*(error_vx);
    INT_vy= INT_vy + 0.01*(error_vy);
    INT_vz= INT_vz + 0.01*(error_vz);
    
    u_dot_d = Kp_vx*(error_vx)   +    Ki_vx*(INT_vx)  +   Kd_vx*(error_vx-error_vx_old);
    v_dot_d = Kp_vy*(error_vy)   +    Ki_vy*(INT_vy)  +   Kd_vy*(error_vy-error_vy_old);
    w_dot_d = Kp_vz*(error_vz)   +    Ki_vz*(INT_vz)  +   Kd_vz*(error_vz-error_vz_old);
    
    error_vx_old=error_vx;
    error_vy_old=error_vy;
    error_vz_old=error_vz;
    
end

if (flag_vertical_landing==1)
    if (one_time_initial_vertical_landing==1)
        X_i_landing=X;
        Y_i_landing=Y;
        Z_i_landing=Z;
        
        X_f_landing=X_i_landing;
        Y_f_landing=Y_i_landing;
        Z_f_landing=0.0;
        
        INT_X=0;INT_Y=0;INT_Z=0;
        INT_vx=0;INT_vy=0;INT_vz=0;
        
        INT_alpha=0;INT_beta=0;
        
        INT_phi=0;INT_theta=0;INT_psi=0;
        INT_p=0;INT_q=0;INT_r=0;
        
        one_time_initial_vertical_landing=0;
        
    end
    X_d=X_f_landing;
    Y_d=Y_f_landing;
    Z_d=Z_i_landing + 2*(Z_f_landing-Z_i_landing)*(t-tf7)/(tf8-tf7) + (Z_i_landing-Z_f_landing)*((t-tf7)^2)/((tf8-tf7)^2) ;
    if t>tf8
       Z_d = Z_f_landing;
    end
    Kp_X=0.1*4.0;           Ki_X= 0.0;                Kd_X=0.0;
    Kp_Y=0.1*4.0;           Ki_Y= 0.0;                Kd_Y=0.0;
    Kp_Z=2.0;               Ki_Z=0.1;                  Kd_Z=0.0;
    
    Kp_vx= 0.1*4.0*3.0;     Ki_vx=0.0;                Kd_vx=0.0;
    Kp_vy= 0.1*4.0*3.0;     Ki_vy=0.0;                Kd_vy=0.0;
    Kp_vz= 6.0;             Ki_vz=0.0*0.001;          Kd_vz=0.0;
    
    
    error_X = (X_d-X);
    error_Y = (Y_d-Y);
    error_Z = (Z_d-Z);
    
    if(lmt_pos==1)
        
        if(abs(error_X)<limit_position_X)
            
            error_X=0.0;
        end
        if(abs(error_Y)<limit_position_Y)
            
            error_Y=0.0;
        end
        if(abs(error_Z)<limit_position_Z)
            
            error_Z=0.0;
        end
    end
    
    INT_X = INT_X + 0.01*(error_X);
    INT_Y = INT_Y + 0.01*(error_Y);
    INT_Z = INT_Z + 0.01*(error_Z);
    
    U_d = Kp_X*(error_X) +  Ki_X*(INT_X) + Kd_X*(error_X-error_X_old);
    V_d = Kp_Y*(error_Y) +  Ki_Y*(INT_Y) + Kd_Y*(error_Y-error_Y_old);
    W_d = Kp_Z*(error_Z) +  Ki_Z*(INT_Z) + Kd_Z*(error_Z-error_Z_old);
    
    temp_3X1=R_v_b*[U_d;V_d;W_d];
    
    u_d=temp_3X1(1);
    v_d=temp_3X1(2);
    w_d=temp_3X1(3);
    error_X_old=error_X;
    error_Y_old=error_Y;
    error_Z_old=error_Z;
    
    error_vx = (u_d-u);
    error_vy = (v_d-v);
    error_vz = (w_d-w);
    
    if(lmt_vel==1)
        if(abs(error_vx)<limit_velocity_vx)
            error_vx=0.0;
        end
        if(abs(error_vy)<limit_velocity_vy)
            error_vy=0.0;
        end
        if(abs(error_vz)<limit_velocity_vz)
            error_vz=0.0;
        end
    end
    
    INT_vx= INT_vx + 0.01*(error_vx);
    INT_vy= INT_vy + 0.01*(error_vy);
    INT_vz= INT_vz + 0.01*(error_vz);
    
    u_dot_d = Kp_vx*(error_vx)   +    Ki_vx*(INT_vx)  +   Kd_vx*(error_vx-error_vx_old);
    v_dot_d = Kp_vy*(error_vy)   +    Ki_vy*(INT_vy)  +   Kd_vy*(error_vy-error_vy_old);
    w_dot_d = Kp_vz*(error_vz)   +    Ki_vz*(INT_vz)  +   Kd_vz*(error_vz-error_vz_old);
    
    error_vx_old=error_vx;
    error_vy_old=error_vy;
    error_vz_old=error_vz;
    
    
end
%%%%%%%%%%%%%%%%%%%%%%%%%%%%%%%%%%%%%%%%%%%%%%%%%%%%%%%%%%%%%%%%%%%%%%%%%%%%%%%%%%%%%%%%%%%%%%%%%%%%%%%%%%%%%%%%%%%%%%%%%%%
%%%%%%%%%%%%%%%%%%%%%%%%%%%%%%%%%%%%%%%%%%%%%%%%%%%%%%%%%%%%%%%%%%%%%%%%%%%%%%%%%%%%%%%%%%%%%%%%%%%%%%%%%%%%%%%%%%%%%%%%%%%
%%%%%%%%%%%%%%%%%%%%%%%%%%%%%%%%%%%%%%%%%%%%%%%%%%%%%%%%%%%%%%%%%%%%%%%%%%%%%%%%%%%%%%%%%%%%%%%%%%%%%%%%%%%%%%%%%%%%%%%%%%%





%%

%
else
    
    %%% write fail_safe modes here



end


if abs(u_dot_d) > 4.0*9.81

u_dot_d = 4.0*9.81*sign(u_dot_d);

INT_vx=0.0;

end

if abs(v_dot_d) > 4.0*9.81

v_dot_d = 4.0*9.81*sign(v_dot_d);

INT_vy=0.0;

end

if abs(w_dot_d) > 4.0*9.81

w_dot_d = 4.0*9.81*sign(w_dot_d);

INT_vz=0.0;
INT_Z=0.0;

end


flags_global(1)=all_initial_check_ok;
flags_global(2)=default_mode;

flags_global(3)=quad_mode;
flags_global(4)=Transition_mode;
flags_global(5)=Fixed_wing_mode;

flags_global(6)=fail_safe_mode;
flags_global(7)=fail_safe_mode_hover;
flags_global(8)=fail_safe_mode_land;
flags_global(9)=fail_safe_mode_2;


flags_global(10)=flag_initial_lift_off_hover;
flags_global(11)=flag_vertical_takeoff;
flags_global(12)=flag_hover_mode;

flags_global(13)=flag_circle_mode;
flags_global(14)=flag_cruise_mode;

flags_global(15)=flag_vertical_landing;

flags_global(16)=one_time_initial_lift_off_hover;
flags_global(17)=one_time_initial_vertical_takeoff;
flags_global(18)=one_time_initial_hover_mode;
flags_global(19)=one_time_initial_cruise_mode;

flags_global(20)=one_time_initial_circle_mode;
flags_global(21)=one_time_initial_vertical_landing;
flags_global(22)=flag_brake_mode;

flags_global(23)=flag_forward_transition;
flags_global(24)=flag_reverse_transition;
flags_global(25)=one_time_initial_flag_forward_transition;
flags_global(26)=one_time_initial_flag_reverse_transition ;


guidance_global(1)=X_i_takeoff;  guidance_global(2)=Y_i_takeoff;  guidance_global(3)=Z_i_takeoff; guidance_global(4)=X_f_takeoff; guidance_global(5)=Y_f_takeoff; guidance_global(6)=Z_f_takeoff;

guidance_global(7)=X_i_hover; guidance_global(8)=Y_i_hover; guidance_global(9)=Z_i_hover; guidance_global(10)=X_f_hover; guidance_global(11)=Y_f_hover;guidance_global(12)=Z_f_hover;

guidance_global(13)=X_i_cruise; guidance_global(14)=Y_i_cruise; guidance_global(15)=Z_i_cruise; guidance_global(16)=X_f_cruise; guidance_global(17)=Y_f_cruise; guidance_global(18)=Z_f_cruise;

guidance_global(19)=X_i_circle; guidance_global(20)=Y_i_circle; guidance_global(21)=Z_i_circle; guidance_global(22)=X_f_circle; guidance_global(23)=Y_f_circle;guidance_global(24)= Z_f_circle;

guidance_global(25)=X_i_landing; guidance_global(26)=Y_i_landing;guidance_global(27)= Z_i_landing; guidance_global(28)=X_f_landing; guidance_global(29)=Y_f_landing; guidance_global(30)=Z_f_landing;

guidance_global(31)=X_f_forward_transition; guidance_global(32)=Y_f_forward_transition; guidance_global(33)=Z_f_forward_transition;

guidance_global(37)=X_i_forward_transition;guidance_global(38)= Y_i_forward_transition; guidance_global(39)=Z_i_forward_transition;

guidance_global(43)=X_f_reverse_transition; guidance_global(44)=Y_f_reverse_transition; guidance_global(45)=Z_f_reverse_transition;

guidance_global(49)=X_i_reverse_transition; guidance_global(50)=Y_i_reverse_transition; guidance_global(51)=Z_i_reverse_transition;

INT_global(1)=INT_X; INT_global(2)=INT_Y; INT_global(3)=INT_Z;

INT_global(4)=INT_vx; INT_global(5)=INT_vy;INT_global(6)= INT_vz;

INT_global(7)=INT_phi; INT_global(8)=INT_theta; INT_global(9)=INT_psi;

INT_global(10)=INT_p; INT_global(11)=INT_q; INT_global(12)=INT_r;

INT_global(13)=INT_alpha; INT_global(14)=INT_beta;

param_guidance(1)=R_circ;
param_guidance(2)=cruise_speed;
param_guidance(3)=lmt_pos; 
param_guidance(4)=lmt_vel;


error_global(1)=error_X_old; error_global(2)=error_Y_old; error_global(3)=error_Z_old;

error_global(4)=error_vx_old; error_global(5)=error_vy_old; error_global(6)=error_vz_old;






end

== matlab function Autopilot_q_full_5may_new/AUTOPILOT /Autopilot Quad mode/Roll Controller/MATLAB Function1 ==
  data: t input; TT input; mass input; a_y_d input; phi_d output
function phi_d  = fcn(t, TT, mass, a_y_d)
TT=sum(TT);
if (abs(TT)<1)
    TT=1;
end
while (abs(mass*a_y_d/TT)) >= 0.7 %% 45 deg max
    TT=TT+1;
end
phi_d=asin((mass/TT)*a_y_d);

end

== matlab function Autopilot_q_full_5may_new/AUTOPILOT /Autopilot Quad mode/Roll Controller/MATLAB Function2 ==
  data: angular_state input; phi_dot_d input; p_d output
function p_d  = fcn(angular_state,phi_dot_d)
p=angular_state(1);
q=angular_state(2);
r=angular_state(3);
phi=angular_state(4);
theta=angular_state(5);
psi=angular_state(6);
p_d= phi_dot_d - q*sin(phi)*tan(theta)-r*cos(phi)*tan(theta);

end

== matlab function Autopilot_q_full_5may_new/AUTOPILOT /Autopilot Quad mode/Pitch Controller/MATLAB Function3 ==
  data: t input; TT input; mass input; a_x_d input; theta_d output
function theta_d  = fcn(t, TT, mass, a_x_d)
TT=sum(TT);
if (abs(TT)<1)
    TT=1;
end
while (abs(mass*a_x_d/TT)) >= 0.7 %% 45 deg max
    TT=TT+1;
end
theta_d=asin(-(mass/TT)*a_x_d);



end

== matlab function Autopilot_q_full_5may_new/AUTOPILOT /Autopilot Quad mode/Pitch Controller/MATLAB Function4 ==
  data: angular_state input; theta_dot_d input; q_d output
function q_d  = fcn(angular_state,theta_dot_d)

p=angular_state(1);
q=angular_state(2);
r=angular_state(3);
phi=angular_state(4);
theta=angular_state(5);
psi=angular_state(6);

if (abs(phi)>(pi/2.5))
		
	q_d=(theta_dot_d +r*sin(phi));
		
else
		
	q_d=(theta_dot_d +r*sin(phi))/cos(phi);
end

end

== matlab function Autopilot_q_full_5may_new/AUTOPILOT /Autopilot Quad mode/Heading Controller/MATLAB Function5 ==
  data: t input; psi_d output; u input; v input; psi_d input
function psi_d  = fcn(t,u,v, psi_d)
psi_d=psi_d;


% if t>=35 && t<60
% psi_d= -(pi/50)*(t-35);
% end
% 
% 
% if t>=60 && t<85
%     psi_d= -(pi/2) - (pi/50)*(t-60);
% end
% 
% if t>=85 && t<110
%     psi_d= (pi) - (pi/50)*(t-85);
% end
% 
% if t>=110 && t<135
%     psi_d= (pi/2) - (pi/50)*(t-110);
% end
    




end

== matlab function Autopilot_q_full_5may_new/AUTOPILOT /Autopilot Quad mode/Heading Controller/MATLAB Function6 ==
  data: angular_state input; psi_dot_d input; r_d output
function r_d  = fcn(angular_state,psi_dot_d)

p=angular_state(1);
q=angular_state(2);
r=angular_state(3);
phi=angular_state(4);
theta=angular_state(5);
psi=angular_state(6);
if (abs(phi)>=((89.0)/57.3))
    phi=abs(phi)*89.0/(57.3*phi);
end
r_d = (psi_dot_d - q*sin(phi)*sec(theta))/(cos(phi)*sec(theta));
end

== matlab function Autopilot_q_full_5may_new/AUTOPILOT /Autopilot Quad mode/Heading Controller/MATLAB Function ==
  data: psi_d input; psi_error output; psi input
function psi_error = fcn(psi_d, psi)

psi_error=psi_d-psi;

if ( abs(psi_error) > pi )
    psi_error = -(psi_error/(abs(psi_error)))*abs((2*pi) - abs(psi_error));
end

end

== matlab function Autopilot_q_full_5may_new/AUTOPILOT /Autopilot Transition mode/Forward transition/Trim setting/MATLAB Function1 ==
  data: aero_data input; structure_data input; V_trim input; alpha_trim output; beta_trim output; delta_e_trim output; delta_a_trim output; delta_r_trim output; Tx_trim output; stall_speed output; propulsion_data input; atmos_data input
function [alpha_trim,beta_trim,delta_e_trim,delta_a_trim,delta_r_trim,Tx_trim,stall_speed]= Autopilot(aero_data,structure_data,V_trim,propulsion_data, atmos_data)
b1=propulsion_data(1); % b and d of vtol propellers
d1=propulsion_data(2);
b1_inv=1.0/b1;
%%
rho=atmos_data(4); % density
%%
V=V_trim;
mass=structure_data(1,1);s=structure_data(1,4);

CLo =aero_data(1,1); CL_alpha=aero_data(1,2);CL_beta=aero_data(1,3); CL_delta_e=aero_data(1,4); CL_delta_a=aero_data(1,5); CL_delta_r=aero_data(1,6); CL_p=aero_data(1,7);CL_q=aero_data(1,8);CL_r=aero_data(1,9);

Cdo =aero_data(2,1); Cd_alpha=aero_data(2,2);Cd_beta=aero_data(2,3); Cd_delta_e=aero_data(2,4); Cd_delta_a=aero_data(2,5); Cd_delta_r=aero_data(2,6); Cd_p=aero_data(2,7);Cd_q=aero_data(2,8);Cd_r=aero_data(2,9);

CYo =aero_data(3,1); CY_alpha=aero_data(3,2);CY_beta=aero_data(3,3); CY_delta_e=aero_data(3,4); CY_delta_a=aero_data(3,5); CY_delta_r=aero_data(3,6); CY_p=aero_data(3,7);CY_q=aero_data(3,8);CY_r=aero_data(3,9);

Clo =aero_data(4,1); Cl_alpha=aero_data(4,2);Cl_beta=aero_data(4,3); Cl_delta_e=aero_data(4,4); Cl_delta_a=aero_data(4,5); Cl_delta_r=aero_data(4,6); Cl_p=aero_data(4,7);Cl_q=aero_data(4,8);Cl_r=aero_data(4,9);

Cmo =aero_data(5,1); Cm_alpha=aero_data(5,2);Cm_beta=aero_data(5,3); Cm_delta_e=aero_data(5,4); Cm_delta_a=aero_data(5,5); Cm_delta_r=aero_data(5,6); Cm_p=aero_data(5,7);Cm_q=aero_data(5,8);Cm_r=aero_data(5,9);

Cno =aero_data(6,1); Cn_alpha=aero_data(6,2);Cn_beta=aero_data(6,3); Cn_delta_e=aero_data(6,4); Cn_delta_a=aero_data(6,5); Cn_delta_r=aero_data(6,6); Cn_p=aero_data(6,7);Cn_q=aero_data(6,8);Cn_r=aero_data(6,9);



g=9.81;



tb=[(mass*g/(0.5*rho*V*V*s)) - CLo;-Cmo];
ta=[CL_alpha,CL_delta_e;Cm_alpha,Cm_delta_e];

trim_set_long = inv(ta)*tb;

alpha_trim = trim_set_long(1);
delta_e_trim = trim_set_long(2);

% CYo + CY_beta*beta + CY_delta_a*delta_a + CY_delta_r*delta_r;
% Clo + Cl_beta*beta + Cl_delta_a*delta_a + Cl_delta_r*delta_r;
% Cno + Cn_beta*beta + Cn_delta_a*delta_a + Cn_delta_r*delta_r;

tb1=[-CYo;-Clo;-Cno];
ta1=[CY_beta,CY_delta_a,CY_delta_r;Cl_beta,Cl_delta_a,Cl_delta_r;Cn_beta,Cn_delta_a,Cn_delta_r];

trim_set_lat=inv(ta1)*tb1;

beta_trim = trim_set_lat(1);
delta_a_trim = trim_set_lat(2);
delta_r_trim = trim_set_lat(3);


% drag = 1/2 *rho *V*V*s*( Cdo + Cd_alpha*alpha + Cd_delta_e*delta_e );
Tx_trim =  0.5*rho*V*V*s*( Cdo + Cd_alpha*alpha_trim + Cd_delta_e*delta_e_trim );

stall_speed=sqrt((mass*g)/(0.5*1.225*s*(CLo+CL_alpha*(12.0/57.3))));
